simulink model "FS_AWD_Working"  (Simulink 10.0)
settings: Solver=ode45  StartTime=0.0  StopTime=inf  RelTol=1e-3  EnableMultiTasking=on
PreLoadFcn:
  | FSE_Parameters
undefined symbols (not defined in the file): i_Diff, TC_Decr_Gas, TC_Derivative, TC_Incr_Gas, TC_On, TC_Relay_Off, TC_Relay_On
libraries: CarMaker4SL x26, simulink x3, simulink_extras x2
(part 2 of 2)

== system FS_AWD_Working/CarMaker/IPG Vehicle/CarAndTrailer/Forces/Vehicle Forces ==
  Sync_In : Inport
  Bus Creator1 : BusCreator  Inputs=12
  Bus Creator8 : BusCreator  Inputs=16
  BusCreator1 : BusCreator  Inputs=4
  BusCreator2 : BusCreator  Inputs=9
  Demux : Demux  Outputs=16
  Demux1 : Demux  Outputs=12
  Demux2 : Demux  Outputs=13
  Forces : S-Function  FunctionName=CM_Sfun  Parameters='Forces'  SFunctionDeploymentMode=off  EnableBusSupport=off
  Terminator : Terminator
  Sync_Out : Outport  VectorParamsAs1DForOutWhenUnconnected=off
  Car.Virtual : Outport  Port=2  VectorParamsAs1DForOutWhenUnconnected=off
  Car.Aero : Outport  Port=3  VectorParamsAs1DForOutWhenUnconnected=off
  Car.Load : Outport  Port=4  VectorParamsAs1DForOutWhenUnconnected=off
  wires:
  BusCreator1/1 -> Terminator/1  "Aero IF (in)"
  Demux2/13 -> BusCreator2/9  "car Aero Trq_1 z"
  Demux2/12 -> BusCreator2/8  "car Aero Trq_1 y"
  Demux2/11 -> BusCreator2/7  "car Aero Trq_1 x"
  Demux2/10 -> BusCreator2/6  "car Aero Frc_1 z"
  Demux2/9 -> BusCreator2/5  "car Aero Frc_1 y"
  Demux2/8 -> BusCreator2/4  "car Aero Frc_1 x"
  Demux2/7 -> BusCreator2/3  "car Aero PoA_1 z"
  Demux2/6 -> BusCreator2/2  "car Aero PoA_1 y"
  Demux2/5 -> BusCreator2/1  "car Aero PoA_1 x"
  Demux2/4 -> BusCreator1/4  "car Aero tau_1"
  Demux2/3 -> BusCreator1/3  "car Aero ApproachVel_1 z"
  Demux2/2 -> BusCreator1/2  "car Aero ApproachVel_1 y"
  Demux2/1 -> BusCreator1/1  "car Aero ApproachVel_1 x"
  Demux/16 -> Bus Creator8/16  "Car Load_3 tz"
  Demux/15 -> Bus Creator8/15  "Car Load_3 ty"
  Demux/14 -> Bus Creator8/14  "Car Load_3 tx"
  Demux/13 -> Bus Creator8/13  "Car Load_3 mass"
  Demux1/12 -> Bus Creator1/12  "Car Virtual Trq_0 z"
  Demux1/11 -> Bus Creator1/11  "Car Virtual Trq_0 y"
  Demux1/10 -> Bus Creator1/10  "Car Virtual Trq_0 x"
  Demux1/9 -> Bus Creator1/9  "Car Virtual Trq_1 z"
  Demux1/8 -> Bus Creator1/8  "Car Virtual Trq_1 y"
  Demux1/7 -> Bus Creator1/7  "Car Virtual Trq_1 x"
  Demux1/6 -> Bus Creator1/6  "Car Virtual Frc_0 z"
  Demux1/5 -> Bus Creator1/5  "Car Virtual Frc_0 y"
  Demux1/4 -> Bus Creator1/4  "Car Virtual Frc_0 x"
  Sync_In/1 -> Forces/1
  Forces/1 -> Sync_Out/1
  BusCreator2/1 -> Car.Aero/1
  Demux1/1 -> Bus Creator1/1  "Car Virtual Frc_1 x"
  Demux1/2 -> Bus Creator1/2  "Car Virtual Frc_1 y"
  Demux1/3 -> Bus Creator1/3  "Car Virtual Frc_1 z"
  Forces/3 -> Demux2/1
  Forces/2 -> Demux1/1
  Bus Creator1/1 -> Car.Virtual/1
  Bus Creator8/1 -> Car.Load/1
  Demux/1 -> Bus Creator8/1  "Car Load_0 mass"
  Demux/2 -> Bus Creator8/2  "Car Load_0 tx"
  Demux/3 -> Bus Creator8/3  "Car Load_0 ty"
  Demux/4 -> Bus Creator8/4  "Car Load_0 tz"
  Demux/5 -> Bus Creator8/5  "Car Load_1 mass"
  Demux/6 -> Bus Creator8/6  "Car Load_1 tx"
  Demux/7 -> Bus Creator8/7  "Car Load_1 ty"
  Demux/8 -> Bus Creator8/8  "Car Load_1 tz"
  Demux/9 -> Bus Creator8/9  "Car Load_2 mass"
  Demux/10 -> Bus Creator8/10  "Car Load_2 tx"
  Demux/11 -> Bus Creator8/11  "Car Load_2 ty"
  Demux/12 -> Bus Creator8/12  "Car Load_2 tz"
  Forces/4 -> Demux/1

== system FS_AWD_Working/CarMaker/IPG Vehicle/CarAndTrailer/Trailer/CreateBus Car.Hitch.FrcTrq ==
  In1 : Inport
  Bus Creator7 : BusCreator  Inputs=6
  Demux7 : Demux  Outputs=6
  Out1 : Outport  VectorParamsAs1DForOutWhenUnconnected=off
  wires:
  In1/1 -> Demux7/1
  Bus Creator7/1 -> Out1/1
  Demux7/6 -> Bus Creator7/6  "Car Hitch Trq2Car z"
  Demux7/5 -> Bus Creator7/5  "Car Hitch Trq2Car y"
  Demux7/4 -> Bus Creator7/4  "Car Hitch Trq2Car x"
  Demux7/3 -> Bus Creator7/3  "Car Hitch Frc2Car z"
  Demux7/2 -> Bus Creator7/2  "Car Hitch Frc2Car y"
  Demux7/1 -> Bus Creator7/1  "Car Hitch Frc2Car x"

== system FS_AWD_Working/CarMaker/IPG Vehicle/CarAndTrailer/Trailer/CreateBus Vhcl.Motion ==
  In1 : Inport
  BusCreator : BusCreator  Inputs=15
  Demux : Demux  Outputs=15
  Out1 : Outport  VectorParamsAs1DForOutWhenUnconnected=off
  wires:
  Demux/15 -> BusCreator/15  "Vhcl YawAcc"
  Demux/14 -> BusCreator/14  "Vhcl YawVel"
  Demux/13 -> BusCreator/13  "Vhcl Yaw"
  Demux/12 -> BusCreator/12  "Vhcl PitchAcc"
  Demux/11 -> BusCreator/11  "Vhcl PitchVel"
  Demux/10 -> BusCreator/10  "Vhcl Pitch"
  Demux/9 -> BusCreator/9  "Vhcl RollAcc"
  Demux/8 -> BusCreator/8  "Vhcl RollVel"
  Demux/7 -> BusCreator/7  "Vhcl Roll"
  Demux/6 -> BusCreator/6  "Vhcl Hitch_Pos z"
  Demux/5 -> BusCreator/5  "Vhcl Hitch_Pos y"
  Demux/4 -> BusCreator/4  "Vhcl Hitch_Pos x"
  Demux/3 -> BusCreator/3  "Vhcl sRoad"
  Demux/2 -> BusCreator/2  "Vhcl Distance"
  Demux/1 -> BusCreator/1  "Vhcl v"
  In1/1 -> Demux/1
  BusCreator/1 -> Out1/1

== system FS_AWD_Working/CarMaker/IPG Vehicle/CarAndTrailer/Trailer/CreateBus Vhcl.PoI ==
  In1 : Inport
  Bus Creator3 : BusCreator  Inputs=18
  Demux3 : Demux  Outputs=18
  Out1 : Outport  VectorParamsAs1DForOutWhenUnconnected=off
  wires:
  Demux3/18 -> Bus Creator3/18  "Vhcl PoI_GCS Elev"
  Demux3/17 -> Bus Creator3/17  "Vhcl PoI_GCS Lat"
  Demux3/16 -> Bus Creator3/16  "Vhcl PoI_GCS Long"
  Demux3/15 -> Bus Creator3/15  "Vhcl PoI_Acc_1 z"
  Demux3/14 -> Bus Creator3/14  "Vhcl PoI_Acc_1 y"
  Demux3/13 -> Bus Creator3/13  "Vhcl PoI_Acc_1 x"
  Demux3/12 -> Bus Creator3/12  "Vhcl PoI_Vel_1 z"
  Demux3/11 -> Bus Creator3/11  "Vhcl PoI_Vel_1 y"
  Demux3/10 -> Bus Creator3/10  "Vhcl PoI_Vel_1 x"
  Demux3/9 -> Bus Creator3/9  "Vhcl PoI_Acc z"
  Demux3/8 -> Bus Creator3/8  "Vhcl PoI_Acc y"
  Demux3/7 -> Bus Creator3/7  "Vhcl PoI_Acc x"
  Demux3/6 -> Bus Creator3/6  "Vhcl PoI_Vel z"
  Demux3/5 -> Bus Creator3/5  "Vhcl PoI_Vel y"
  Demux3/4 -> Bus Creator3/4  "Vhcl PoI_Vel x"
  Demux3/3 -> Bus Creator3/3  "Vhcl PoI_Pos z"
  Demux3/2 -> Bus Creator3/2  "Vhcl PoI_Pos y"
  In1/1 -> Demux3/1
  Bus Creator3/1 -> Out1/1
  Demux3/1 -> Bus Creator3/1  "Vhcl PoI_Pos x"

== system FS_AWD_Working/CarMaker/IPG Vehicle/CarAndTrailer/Trailer/CreateBus Vhcl.Steering ==
  In1 : Inport
  Bus Creator3 : BusCreator  Inputs=4
  Demux : Demux
  Out1 : Outport  VectorParamsAs1DForOutWhenUnconnected=off
  wires:
  Bus Creator3/1 -> Out1/1
  Demux/1 -> Bus Creator3/1  "Vhcl Steering Ang"
  Demux/3 -> Bus Creator3/3  "Vhcl Steering AngAcc"
  Demux/2 -> Bus Creator3/2  "Vhcl Steering AngVel"
  Demux/4 -> Bus Creator3/4  "Vhcl Steering Trq"
  In1/1 -> Demux/1

== system FS_AWD_Working/CarMaker/IPG Vehicle/CarAndTrailer/Trailer/CreateBus Vhcl.Wheel.FL ==
  In1 : Inport
  Bus Creator3 : BusCreator  Inputs=14
  Demux3 : Demux  Outputs=14
  Out1 : Outport  VectorParamsAs1DForOutWhenUnconnected=off
  wires:
  Demux3/14 -> Bus Creator3/14  "Vhcl Wheel FL Trq_WhlBearing"
  Demux3/13 -> Bus Creator3/13  "Vhcl Wheel FL Trq_T2W"
  Demux3/12 -> Bus Creator3/12  "Vhcl Wheel FL SideSlip"
  Demux3/11 -> Bus Creator3/11  "Vhcl Wheel FL LongSlip"
  Demux3/10 -> Bus Creator3/10  "Vhcl Wheel FL vBelt"
  Demux3/9 -> Bus Creator3/9  "Vhcl Wheel FL Fz"
  Demux3/8 -> Bus Creator3/8  "Vhcl Wheel FL Fy"
  Demux3/7 -> Bus Creator3/7  "Vhcl Wheel FL Fx"
  Demux3/6 -> Bus Creator3/6  "Vhcl Wheel FL r_zxy z"
  Demux3/5 -> Bus Creator3/5  "Vhcl Wheel FL r_zxy y"
  Demux3/4 -> Bus Creator3/4  "Vhcl Wheel FL r_zxy x"
  Demux3/3 -> Bus Creator3/3  "Vhcl Wheel FL t z"
  Demux3/2 -> Bus Creator3/2  "Vhcl Wheel FL t y"
  In1/1 -> Demux3/1
  Bus Creator3/1 -> Out1/1
  Demux3/1 -> Bus Creator3/1  "Vhcl Wheel FL t x"

== system FS_AWD_Working/CarMaker/IPG Vehicle/CarAndTrailer/Trailer/CreateBus Vhcl.Wheel.FR ==
  In1 : Inport
  Bus Creator3 : BusCreator  Inputs=14
  Demux3 : Demux  Outputs=14
  Out1 : Outport  VectorParamsAs1DForOutWhenUnconnected=off
  wires:
  Demux3/14 -> Bus Creator3/14  "Vhcl Wheel FR Trq_WhlBearing"
  Demux3/13 -> Bus Creator3/13  "Vhcl Wheel FR Trq_T2W"
  Demux3/12 -> Bus Creator3/12  "Vhcl Wheel FR SideSlip"
  Demux3/11 -> Bus Creator3/11  "Vhcl Wheel FR LongSlip"
  Demux3/10 -> Bus Creator3/10  "Vhcl Wheel FR vBelt"
  Demux3/9 -> Bus Creator3/9  "Vhcl Wheel FR Fz"
  Demux3/8 -> Bus Creator3/8  "Vhcl Wheel FR Fy"
  Demux3/7 -> Bus Creator3/7  "Vhcl Wheel FR Fx"
  Demux3/6 -> Bus Creator3/6  "Vhcl Wheel FR r_zxy z"
  Demux3/5 -> Bus Creator3/5  "Vhcl Wheel FR r_zxy y"
  Demux3/4 -> Bus Creator3/4  "Vhcl Wheel FR r_zxy x"
  Demux3/3 -> Bus Creator3/3  "Vhcl Wheel FR t z"
  Demux3/2 -> Bus Creator3/2  "Vhcl Wheel FR t y"
  In1/1 -> Demux3/1
  Bus Creator3/1 -> Out1/1
  Demux3/1 -> Bus Creator3/1  "Vhcl Wheel FR t x"

== system FS_AWD_Working/CarMaker/IPG Vehicle/CarAndTrailer/Trailer/CreateBus Vhcl.Wheel.RL ==
  In1 : Inport
  Bus Creator3 : BusCreator  Inputs=14
  Demux3 : Demux  Outputs=14
  Out1 : Outport  VectorParamsAs1DForOutWhenUnconnected=off
  wires:
  Demux3/14 -> Bus Creator3/14  "Vhcl Wheel RL Trq_WhlBearing"
  Demux3/13 -> Bus Creator3/13  "Vhcl Wheel RL Trq_T2W"
  Demux3/12 -> Bus Creator3/12  "Vhcl Wheel RL SideSlip"
  Demux3/11 -> Bus Creator3/11  "Vhcl Wheel RL LongSlip"
  Demux3/10 -> Bus Creator3/10  "Vhcl Wheel RL vBelt"
  Demux3/9 -> Bus Creator3/9  "Vhcl Wheel RL Fz"
  Demux3/8 -> Bus Creator3/8  "Vhcl Wheel RL Fy"
  Demux3/7 -> Bus Creator3/7  "Vhcl Wheel RL Fx"
  Demux3/6 -> Bus Creator3/6  "Vhcl Wheel RL r_zxy z"
  Demux3/5 -> Bus Creator3/5  "Vhcl Wheel RL r_zxy y"
  Demux3/4 -> Bus Creator3/4  "Vhcl Wheel RL r_zxy x"
  Demux3/3 -> Bus Creator3/3  "Vhcl Wheel RL t z"
  Demux3/2 -> Bus Creator3/2  "Vhcl Wheel RL t y"
  In1/1 -> Demux3/1
  Bus Creator3/1 -> Out1/1
  Demux3/1 -> Bus Creator3/1  "Vhcl Wheel RL t x"

== system FS_AWD_Working/CarMaker/IPG Vehicle/CarAndTrailer/Trailer/CreateBus Vhcl.Wheel.RR ==
  In1 : Inport
  Bus Creator3 : BusCreator  Inputs=14
  Demux3 : Demux  Outputs=14
  Out1 : Outport  VectorParamsAs1DForOutWhenUnconnected=off
  wires:
  Demux3/14 -> Bus Creator3/14  "Vhcl Wheel RR Trq_WhlBearing"
  Demux3/13 -> Bus Creator3/13  "Vhcl Wheel RR Trq_T2W"
  Demux3/12 -> Bus Creator3/12  "Vhcl Wheel RR SideSlip"
  Demux3/11 -> Bus Creator3/11  "Vhcl Wheel RR LongSlip"
  Demux3/10 -> Bus Creator3/10  "Vhcl Wheel RR vBelt"
  Demux3/9 -> Bus Creator3/9  "Vhcl Wheel RR Fz"
  Demux3/8 -> Bus Creator3/8  "Vhcl Wheel RR Fy"
  Demux3/7 -> Bus Creator3/7  "Vhcl Wheel RR Fx"
  Demux3/6 -> Bus Creator3/6  "Vhcl Wheel RR r_zxy z"
  Demux3/5 -> Bus Creator3/5  "Vhcl Wheel RR r_zxy y"
  Demux3/4 -> Bus Creator3/4  "Vhcl Wheel RR r_zxy x"
  Demux3/3 -> Bus Creator3/3  "Vhcl Wheel RR t z"
  Demux3/2 -> Bus Creator3/2  "Vhcl Wheel RR t y"
  In1/1 -> Demux3/1
  Bus Creator3/1 -> Out1/1
  Demux3/1 -> Bus Creator3/1  "Vhcl Wheel RR t x"

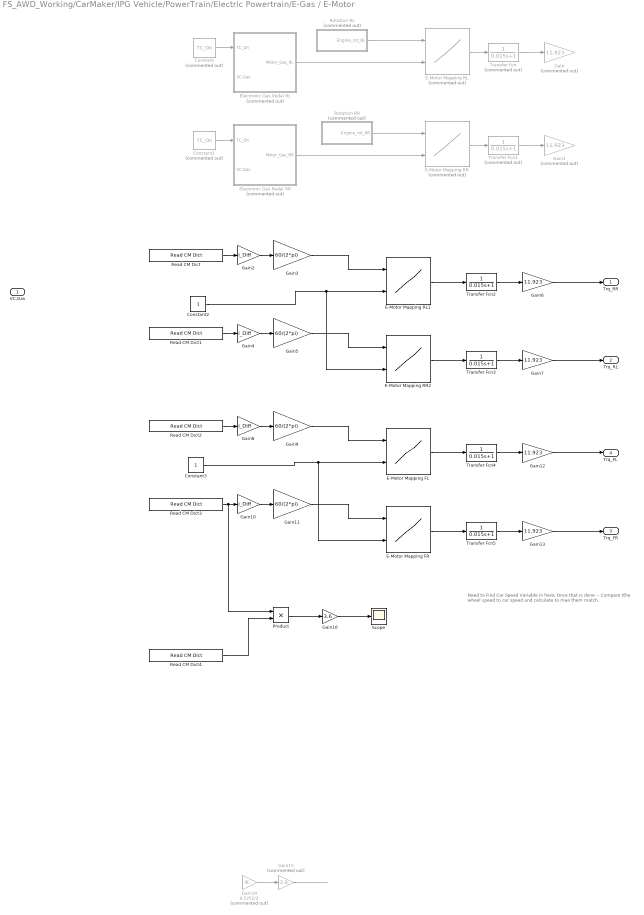
== system FS_AWD_Working/CarMaker/IPG Vehicle/PowerTrain/Electric Powertrain/E-Gas / E-Motor ==
  note: Need to Find Car Speed Variable in here;
      | Once that is done --
      | Compare tthe wheel speed to car speed and calculate to mae them match.
  VC.Gas : Inport
  Constant : Constant  Commented=on  Value=TC_On
  Constant1 : Constant  Commented=on  Value=TC_On
  Constant2 : Constant
  Constant3 : Constant
  E-Motor Mapping FL : Lookup2D  RowIndex=AMKData_GC(1,2:end)  ColumnIndex=AMKData_GC(2:end,1)  Table=AMKData_GC(2:end,2:end)'  LookUpMeth=Interpolation-Use End Values
  E-Motor Mapping FR : Lookup2D  RowIndex=AMKData_GC(1,2:end)  ColumnIndex=AMKData_GC(2:end,1)  Table=AMKData_GC(2:end,2:end)'  LookUpMeth=Interpolation-Use End Values
  E-Motor Mapping RL : Lookup2D  Commented=on  RowIndex=FSE_M120(1,2:end)  ColumnIndex=FSE_M120(2:end,1)  Table=FSE_M120(2:end,2:end)'  LookUpMeth=Interpolation-Use End Values
  E-Motor Mapping RL1 : Lookup2D  RowIndex=AMKData_GC(1,2:end)  ColumnIndex=AMKData_GC(2:end,1)  Table=AMKData_GC(2:end,2:end)'  LookUpMeth=Interpolation-Use End Values
  E-Motor Mapping RR : Lookup2D  Commented=on  RowIndex=FSE_M120(1,2:end)  ColumnIndex=FSE_M120(2:end,1)  Table=FSE_M120(2:end,2:end)'  LookUpMeth=Interpolation-Use End Values
  E-Motor Mapping RR2 : Lookup2D  RowIndex=AMKData_GC(1,2:end)  ColumnIndex=AMKData_GC(2:end,1)  Table=AMKData_GC(2:end,2:end)'  LookUpMeth=Interpolation-Use End Values
  Electronic Gas Pedal RL : Subsystem  Commented=on
  Electronic Gas Pedal RR : Subsystem  Commented=on
  Gain : Gain  Commented=on  Gain=11.923
  Gain1 : Gain  Commented=on  Gain=11.923
  Gain{2,4,8,10} (4 alike) : Gain  Gain=i_Diff
  Gain{3,5,9,11} (4 alike) : Gain  Gain=60/(2*pi)
  Gain{6..7,12..13} (4 alike) : Gain  Gain=11.923
  Gain14 : Gain  Commented=on  Gain=0.5252/2
  Gain15 : Gain  Commented=on  Gain=3.6
  Gain16 : Gain  Gain=3.6
  Product : Product
  Read CM Dict : CarMaker4SL/Read CM Dict  xname=Car.WheelSpd_RR  xsync=off
  Read CM Dict1 : CarMaker4SL/Read CM Dict  xname=Car.WheelSpd_RL  xsync=off
  Read CM Dict2 : CarMaker4SL/Read CM Dict  xname=Car.WheelSpd_FL  xsync=off
  Read CM Dict3 : CarMaker4SL/Read CM Dict  xname=Car.WheelSpd_FR  xsync=off
  Read CM Dict4 : CarMaker4SL/Read CM Dict  xname=Car.WFL.Radius  xsync=off
  Rotation RL : Subsystem  Commented=on
  Rotation RR : Subsystem  Commented=on
  Scope : Scope
  Transfer Fcn : TransferFcn  Commented=on  Denominator=[0.015 1]
  Transfer Fcn1 : TransferFcn  Commented=on  Denominator=[0.015 1]
  Transfer Fcn{2..5} (4 alike) : TransferFcn  Denominator=[0.015 1]
  Trq_RR : Outport  VectorParamsAs1DForOutWhenUnconnected=off
  Trq_RL : Outport  Port=2  VectorParamsAs1DForOutWhenUnconnected=off
  Trq_FR : Outport  Port=3  VectorParamsAs1DForOutWhenUnconnected=off
  Trq_FL : Outport  Port=4  VectorParamsAs1DForOutWhenUnconnected=off
  wires:
  Rotation RL/1(Engine_rot_RL) -> E-Motor Mapping RL/1
  Constant/1 -> Electronic Gas Pedal RL/1(TC_On)
  Electronic Gas Pedal RL/1(Motor_Gas_RL) -> E-Motor Mapping RL/2
  Constant1/1 -> Electronic Gas Pedal RR/1(TC_On)
  E-Motor Mapping RL/1 -> Transfer Fcn/1
  Transfer Fcn/1 -> Gain/1
  Rotation RR/1(Engine_rot_RR) -> E-Motor Mapping RR/1
  Electronic Gas Pedal RR/1(Motor_Gas_RR) -> E-Motor Mapping RR/2
  Transfer Fcn1/1 -> Gain1/1
  E-Motor Mapping RR/1 -> Transfer Fcn1/1
  Read CM Dict/1 -> Gain2/1
  Gain2/1 -> Gain3/1
  Gain3/1 -> E-Motor Mapping RL1/1
  Read CM Dict1/1 -> Gain4/1
  Gain4/1 -> Gain5/1
  Gain5/1 -> E-Motor Mapping RR2/1
  Transfer Fcn3/1 -> Gain7/1
  Transfer Fcn2/1 -> Gain6/1
  E-Motor Mapping RL1/1 -> Transfer Fcn2/1
  Gain6/1 -> Trq_RR/1
  Gain7/1 -> Trq_RL/1
  E-Motor Mapping RR2/1 -> Transfer Fcn3/1
  Gain9/1 -> E-Motor Mapping FL/1
  Transfer Fcn5/1 -> Gain13/1
  Transfer Fcn4/1 -> Gain12/1
  Gain12/1 -> Trq_FL/1
  Gain13/1 -> Trq_FR/1
  E-Motor Mapping FL/1 -> Transfer Fcn4/1
  Read CM Dict3/1 -> Product/1, Gain10/1
  Gain10/1 -> Gain11/1
  Gain8/1 -> Gain9/1
  E-Motor Mapping FR/1 -> Transfer Fcn5/1
  Read CM Dict2/1 -> Gain8/1
  Gain11/1 -> E-Motor Mapping FR/1
  Gain14/1 -> Gain15/1
  Gain15/1 -> ?
  Read CM Dict4/1 -> Product/2
  Product/1 -> Gain16/1
  Gain16/1 -> Scope/1
  Constant2/1 -> E-Motor Mapping RR2/2, E-Motor Mapping RL1/2
  Constant3/1 -> E-Motor Mapping FR/2, E-Motor Mapping FL/2

== system FS_AWD_Working/CarMaker/IPG Vehicle/PowerTrain/Electric Powertrain/Gas Pedal ==
  Clock : Clock
  Constant : Constant  Value=0
  Constant1 : Constant
  Fcn : Fcn  Commented=through  Expr=u==0
  Read CM Dict : CarMaker4SL/Read CM Dict  xname=Vhcl.Ignition  xsync=off
  Read CM Dict2 : CarMaker4SL/Read CM Dict  xname=VC.Gas  xsync=off
  Switch : Switch
  Switch1 : Switch
  Write CM Dict : CarMaker4SL/Write CM Dict  xname=Vhcl.Ignition  xsync=off
  VC.Gas : Outport  VectorParamsAs1DForOutWhenUnconnected=off
  wires:
  Read CM Dict2/1 -> Switch/1
  Switch/1 -> VC.Gas/1
  Constant/1 -> Switch/3
  Switch1/1 -> Switch/2, Write CM Dict/1
  Read CM Dict/1 -> Switch1/3
  Constant1/1 -> Switch1/1
  Fcn/1 -> Switch1/2
  Clock/1 -> Fcn/1

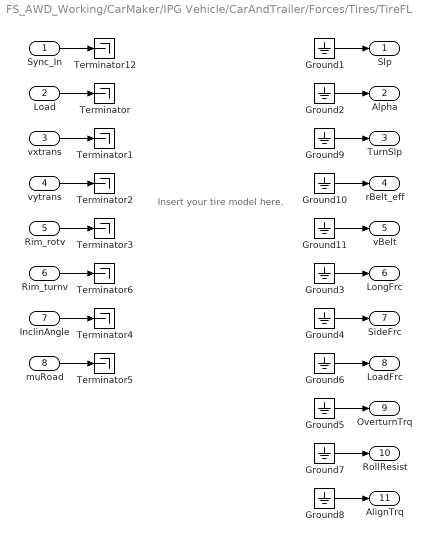
== system FS_AWD_Working/CarMaker/IPG Vehicle/CarAndTrailer/Forces/Tires/TireFL ==
  note: Insert your tire model here.
  Sync_In : Inport
  Load : Inport  Port=2
  vxtrans : Inport  Port=3
  vytrans : Inport  Port=4
  Rim_rotv : Inport  Port=5
  Rim_turnv : Inport  Port=6
  InclinAngle : Inport  Port=7
  muRoad : Inport  Port=8
  Ground{1..11} (11 alike) : Ground
  Terminator{,1..6,12} (8 alike) : Terminator
  Slp : Outport  VectorParamsAs1DForOutWhenUnconnected=off
  Alpha : Outport  Port=2  VectorParamsAs1DForOutWhenUnconnected=off
  TurnSlp : Outport  Port=3  VectorParamsAs1DForOutWhenUnconnected=off
  rBelt_eff : Outport  Port=4  VectorParamsAs1DForOutWhenUnconnected=off
  vBelt : Outport  Port=5  VectorParamsAs1DForOutWhenUnconnected=off
  LongFrc : Outport  Port=6  VectorParamsAs1DForOutWhenUnconnected=off
  SideFrc : Outport  Port=7  VectorParamsAs1DForOutWhenUnconnected=off
  LoadFrc : Outport  Port=8  VectorParamsAs1DForOutWhenUnconnected=off
  OverturnTrq : Outport  Port=9  VectorParamsAs1DForOutWhenUnconnected=off
  RollResist : Outport  Port=10  VectorParamsAs1DForOutWhenUnconnected=off
  AlignTrq : Outport  Port=11  VectorParamsAs1DForOutWhenUnconnected=off
  wires:
  Ground11/1 -> vBelt/1
  Ground10/1 -> rBelt_eff/1
  Ground9/1 -> TurnSlp/1
  Rim_turnv/1 -> Terminator6/1
  Sync_In/1 -> Terminator12/1
  Ground2/1 -> Alpha/1
  Ground3/1 -> LongFrc/1
  Ground4/1 -> SideFrc/1
  Ground5/1 -> OverturnTrq/1
  vxtrans/1 -> Terminator1/1
  vytrans/1 -> Terminator2/1
  Rim_rotv/1 -> Terminator3/1
  InclinAngle/1 -> Terminator4/1
  muRoad/1 -> Terminator5/1
  Load/1 -> Terminator/1
  Ground1/1 -> Slp/1
  Ground6/1 -> LoadFrc/1
  Ground7/1 -> RollResist/1
  Ground8/1 -> AlignTrq/1

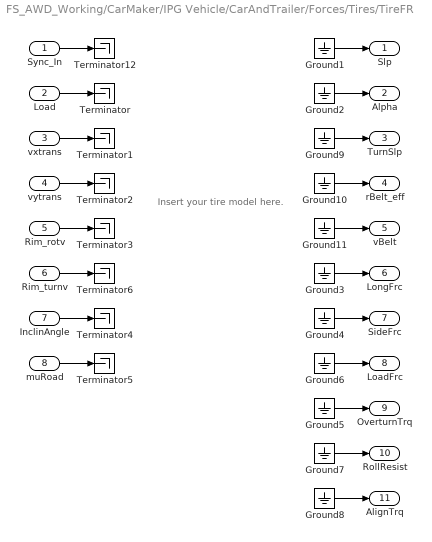
== system FS_AWD_Working/CarMaker/IPG Vehicle/CarAndTrailer/Forces/Tires/TireFR ==
  note: Insert your tire model here.
  Sync_In : Inport
  Load : Inport  Port=2
  vxtrans : Inport  Port=3
  vytrans : Inport  Port=4
  Rim_rotv : Inport  Port=5
  Rim_turnv : Inport  Port=6
  InclinAngle : Inport  Port=7
  muRoad : Inport  Port=8
  Ground{1..11} (11 alike) : Ground
  Terminator{,1..6,12} (8 alike) : Terminator
  Slp : Outport  VectorParamsAs1DForOutWhenUnconnected=off
  Alpha : Outport  Port=2  VectorParamsAs1DForOutWhenUnconnected=off
  TurnSlp : Outport  Port=3  VectorParamsAs1DForOutWhenUnconnected=off
  rBelt_eff : Outport  Port=4  VectorParamsAs1DForOutWhenUnconnected=off
  vBelt : Outport  Port=5  VectorParamsAs1DForOutWhenUnconnected=off
  LongFrc : Outport  Port=6  VectorParamsAs1DForOutWhenUnconnected=off
  SideFrc : Outport  Port=7  VectorParamsAs1DForOutWhenUnconnected=off
  LoadFrc : Outport  Port=8  VectorParamsAs1DForOutWhenUnconnected=off
  OverturnTrq : Outport  Port=9  VectorParamsAs1DForOutWhenUnconnected=off
  RollResist : Outport  Port=10  VectorParamsAs1DForOutWhenUnconnected=off
  AlignTrq : Outport  Port=11  VectorParamsAs1DForOutWhenUnconnected=off
  wires:
  Ground11/1 -> vBelt/1
  Ground10/1 -> rBelt_eff/1
  Ground9/1 -> TurnSlp/1
  Rim_turnv/1 -> Terminator6/1
  Sync_In/1 -> Terminator12/1
  Ground2/1 -> Alpha/1
  Ground3/1 -> LongFrc/1
  Ground4/1 -> SideFrc/1
  Ground5/1 -> OverturnTrq/1
  vxtrans/1 -> Terminator1/1
  vytrans/1 -> Terminator2/1
  Rim_rotv/1 -> Terminator3/1
  InclinAngle/1 -> Terminator4/1
  muRoad/1 -> Terminator5/1
  Load/1 -> Terminator/1
  Ground1/1 -> Slp/1
  Ground6/1 -> LoadFrc/1
  Ground7/1 -> RollResist/1
  Ground8/1 -> AlignTrq/1

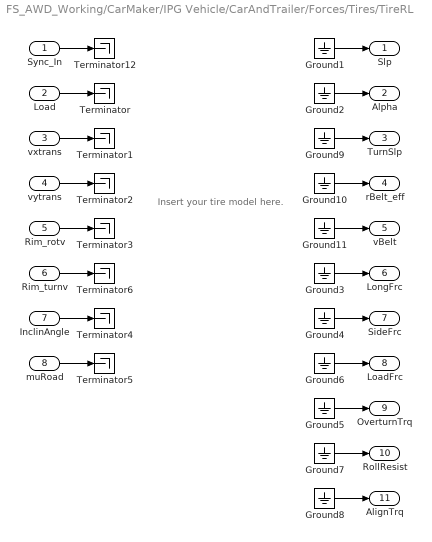
== system FS_AWD_Working/CarMaker/IPG Vehicle/CarAndTrailer/Forces/Tires/TireRL ==
  note: Insert your tire model here.
  Sync_In : Inport
  Load : Inport  Port=2
  vxtrans : Inport  Port=3
  vytrans : Inport  Port=4
  Rim_rotv : Inport  Port=5
  Rim_turnv : Inport  Port=6
  InclinAngle : Inport  Port=7
  muRoad : Inport  Port=8
  Ground{1..11} (11 alike) : Ground
  Terminator{,1..6,12} (8 alike) : Terminator
  Slp : Outport  VectorParamsAs1DForOutWhenUnconnected=off
  Alpha : Outport  Port=2  VectorParamsAs1DForOutWhenUnconnected=off
  TurnSlp : Outport  Port=3  VectorParamsAs1DForOutWhenUnconnected=off
  rBelt_eff : Outport  Port=4  VectorParamsAs1DForOutWhenUnconnected=off
  vBelt : Outport  Port=5  VectorParamsAs1DForOutWhenUnconnected=off
  LongFrc : Outport  Port=6  VectorParamsAs1DForOutWhenUnconnected=off
  SideFrc : Outport  Port=7  VectorParamsAs1DForOutWhenUnconnected=off
  LoadFrc : Outport  Port=8  VectorParamsAs1DForOutWhenUnconnected=off
  OverturnTrq : Outport  Port=9  VectorParamsAs1DForOutWhenUnconnected=off
  RollResist : Outport  Port=10  VectorParamsAs1DForOutWhenUnconnected=off
  AlignTrq : Outport  Port=11  VectorParamsAs1DForOutWhenUnconnected=off
  wires:
  Ground11/1 -> vBelt/1
  Ground10/1 -> rBelt_eff/1
  Ground9/1 -> TurnSlp/1
  Rim_turnv/1 -> Terminator6/1
  Sync_In/1 -> Terminator12/1
  Ground2/1 -> Alpha/1
  Ground3/1 -> LongFrc/1
  Ground4/1 -> SideFrc/1
  Ground5/1 -> OverturnTrq/1
  vxtrans/1 -> Terminator1/1
  vytrans/1 -> Terminator2/1
  Rim_rotv/1 -> Terminator3/1
  InclinAngle/1 -> Terminator4/1
  muRoad/1 -> Terminator5/1
  Load/1 -> Terminator/1
  Ground1/1 -> Slp/1
  Ground6/1 -> LoadFrc/1
  Ground7/1 -> RollResist/1
  Ground8/1 -> AlignTrq/1

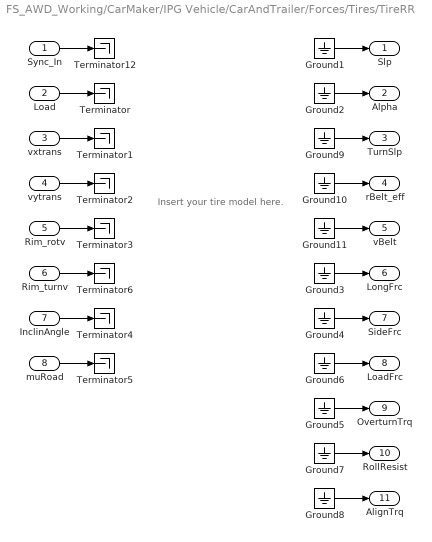
== system FS_AWD_Working/CarMaker/IPG Vehicle/CarAndTrailer/Forces/Tires/TireRR ==
  note: Insert your tire model here.
  Sync_In : Inport
  Load : Inport  Port=2
  vxtrans : Inport  Port=3
  vytrans : Inport  Port=4
  Rim_rotv : Inport  Port=5
  Rim_turnv : Inport  Port=6
  InclinAngle : Inport  Port=7
  muRoad : Inport  Port=8
  Ground{1..11} (11 alike) : Ground
  Terminator{,1..6,12} (8 alike) : Terminator
  Slp : Outport  VectorParamsAs1DForOutWhenUnconnected=off
  Alpha : Outport  Port=2  VectorParamsAs1DForOutWhenUnconnected=off
  TurnSlp : Outport  Port=3  VectorParamsAs1DForOutWhenUnconnected=off
  rBelt_eff : Outport  Port=4  VectorParamsAs1DForOutWhenUnconnected=off
  vBelt : Outport  Port=5  VectorParamsAs1DForOutWhenUnconnected=off
  LongFrc : Outport  Port=6  VectorParamsAs1DForOutWhenUnconnected=off
  SideFrc : Outport  Port=7  VectorParamsAs1DForOutWhenUnconnected=off
  LoadFrc : Outport  Port=8  VectorParamsAs1DForOutWhenUnconnected=off
  OverturnTrq : Outport  Port=9  VectorParamsAs1DForOutWhenUnconnected=off
  RollResist : Outport  Port=10  VectorParamsAs1DForOutWhenUnconnected=off
  AlignTrq : Outport  Port=11  VectorParamsAs1DForOutWhenUnconnected=off
  wires:
  Ground11/1 -> vBelt/1
  Ground10/1 -> rBelt_eff/1
  Ground9/1 -> TurnSlp/1
  Rim_turnv/1 -> Terminator6/1
  Sync_In/1 -> Terminator12/1
  Ground2/1 -> Alpha/1
  Ground3/1 -> LongFrc/1
  Ground4/1 -> SideFrc/1
  Ground5/1 -> OverturnTrq/1
  vxtrans/1 -> Terminator1/1
  vytrans/1 -> Terminator2/1
  Rim_rotv/1 -> Terminator3/1
  InclinAngle/1 -> Terminator4/1
  muRoad/1 -> Terminator5/1
  Load/1 -> Terminator/1
  Ground1/1 -> Slp/1
  Ground6/1 -> LoadFrc/1
  Ground7/1 -> RollResist/1
  Ground8/1 -> AlignTrq/1

== system FS_AWD_Working/CarMaker/IPG Vehicle/PowerTrain/Electric Powertrain/E-Gas / E-Motor/Electronic Gas Pedal RL ==
  TC_On : Inport
  VC.Gas : Inport  Port=2
  Define CM Dict : CarMaker4SL/Define CM Dict  xname=E_Gas_RL  xmono=off  xtype=Double4  xdvaplace=None  xnstates=0  xfirststate=0  xinitial=0
  Read CM Dict1 : CarMaker4SL/Read CM Dict  xname=E_Gas_RL  xsync=off
  Read CM Dict2 : CarMaker4SL/Read CM Dict  xname=Car.LongSlipRL  xsync=off
  Scope : Scope
  Subsystem1 : Subsystem
  Switch : Switch
  Write CM Dict : CarMaker4SL/Write CM Dict  xname=E_Gas_RL  xsync=off
  Motor_Gas_RL : Outport  VectorParamsAs1DForOutWhenUnconnected=off
  wires:
  VC.Gas/1 -> Switch/3, Subsystem1/1(VC.Gas)
  Switch/1 -> Motor_Gas_RL/1
  TC_On/1 -> Switch/2
  Subsystem1/1(E_Gas) -> Write CM Dict/1, Switch/1
  Read CM Dict1/1 -> Subsystem1/2(E_Gas.)
  Read CM Dict2/1 -> Scope/1, Subsystem1/3(Car.LongSlip)

== system FS_AWD_Working/CarMaker/IPG Vehicle/PowerTrain/Electric Powertrain/E-Gas / E-Motor/Electronic Gas Pedal RR ==
  TC_On : Inport
  VC.Gas : Inport  Port=2
  Define CM Dict : CarMaker4SL/Define CM Dict  xname=E_Gas_RR  xmono=off  xtype=Double4  xdvaplace=None  xnstates=0  xfirststate=0  xinitial=0
  Read CM Dict1 : CarMaker4SL/Read CM Dict  xname=E_Gas_RR  xsync=off
  Read CM Dict2 : CarMaker4SL/Read CM Dict  xname=Car.LongSlipRR  xsync=off
  Subsystem1 : Subsystem
  Switch : Switch
  Write CM Dict : CarMaker4SL/Write CM Dict  xname=E_Gas_RR  xsync=off
  Motor_Gas_RR : Outport  VectorParamsAs1DForOutWhenUnconnected=off
  wires:
  TC_On/1 -> Switch/2
  Switch/1 -> Motor_Gas_RR/1
  VC.Gas/1 -> Switch/3, Subsystem1/1(VC.Gas)
  Subsystem1/1(E_Gas) -> Write CM Dict/1, Switch/1
  Read CM Dict2/1 -> Subsystem1/3(Car.LongSlip)
  Read CM Dict1/1 -> Subsystem1/2(E_Gas.)

== system FS_AWD_Working/CarMaker/IPG Vehicle/PowerTrain/Electric Powertrain/E-Gas / E-Motor/Rotation RL ==
  Gain : Gain  Gain=i_Diff
  Gain1 : Gain  Gain=60/(2*pi)
  Read CM Dict : CarMaker4SL/Read CM Dict  xname=Car.WheelSpd_RL  xsync=off
  Engine_rot_RL : Outport  VectorParamsAs1DForOutWhenUnconnected=off
  wires:
  Read CM Dict/1 -> Gain/1
  Gain/1 -> Gain1/1
  Gain1/1 -> Engine_rot_RL/1

== system FS_AWD_Working/CarMaker/IPG Vehicle/PowerTrain/Electric Powertrain/E-Gas / E-Motor/Rotation RR ==
  Gain : Gain  Gain=i_Diff
  Gain1 : Gain  Gain=60/(2*pi)
  Read CM Dict : CarMaker4SL/Read CM Dict  xname=Car.WheelSpd_RR  xsync=off
  Engine_rot_RR : Outport  VectorParamsAs1DForOutWhenUnconnected=off
  wires:
  Gain1/1 -> Engine_rot_RR/1
  Gain/1 -> Gain1/1
  Read CM Dict/1 -> Gain/1

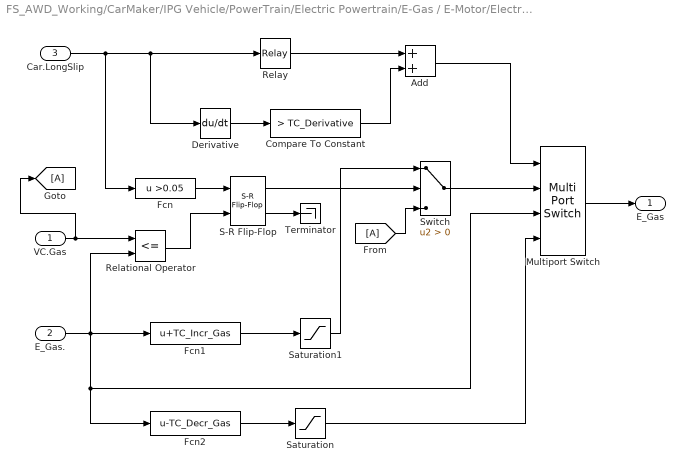
== system FS_AWD_Working/CarMaker/IPG Vehicle/PowerTrain/Electric Powertrain/E-Gas / E-Motor/Electronic Gas Pedal RL/Subsystem1 ==
  VC.Gas : Inport
  E_Gas. : Inport  Port=2
  Car.LongSlip : Inport  Port=3
  Add : Sum
  Compare To Constant : simulink/Logic and Bit Operations/Compare To Constant  relop=>  const=TC_Derivative  OutDataTypeStr=uint8  ZeroCross=off
  Derivative : Derivative
  Fcn : Fcn  Expr=u >0.05
  Fcn1 : Fcn  Expr=u+TC_Incr_Gas
  Fcn2 : Fcn  Expr=u-TC_Decr_Gas
  Multiport Switch : MultiPortSwitch  DataPortOrder=Zero-based contiguous  zeroidx=on
  Relational Operator : RelationalOperator  Operator=<=  RndMeth=Nearest
  Relay : Relay  OnSwitchValue=TC_Relay_On  OffSwitchValue=TC_Relay_Off
  S-R Flip-Flop : simulink_extras/Flip Flops/S-R Flip-Flop  initial_condition=0
  Saturation : Saturate  UpperLimit=1  LowerLimit=0
  Saturation1 : Saturate  UpperLimit=1  LowerLimit=0
  Switch : Switch  Criteria=u2 > Threshold
  Terminator : Terminator
  E_Gas : Outport  VectorParamsAs1DForOutWhenUnconnected=off
  wires:
  Car.LongSlip/1 -> Relay/1, Derivative/1, Fcn/1
  Relay/1 -> Add/1
  Derivative/1 -> Compare To Constant/1
  Compare To Constant/1 -> Add/2
  Add/1 -> Multiport Switch/1
  Multiport Switch/1 -> E_Gas/1
  VC.Gas/1 -> Relational Operator/1, [A]
  E_Gas./1 -> Relational Operator/2, Fcn1/1, Fcn2/1, Multiport Switch/3
  S-R Flip-Flop/2 -> Terminator/1
  S-R Flip-Flop/1 -> Switch/2
  Switch/1 -> Multiport Switch/2
  Fcn/1 -> S-R Flip-Flop/1
  Relational Operator/1 -> S-R Flip-Flop/2
  Fcn1/1 -> Saturation1/1
  Saturation1/1 -> Switch/1
  Fcn2/1 -> Saturation/1
  Saturation/1 -> Multiport Switch/4
  [A] -> Switch/3

== system FS_AWD_Working/CarMaker/IPG Vehicle/PowerTrain/Electric Powertrain/E-Gas / E-Motor/Electronic Gas Pedal RR/Subsystem1 ==
  VC.Gas : Inport
  E_Gas. : Inport  Port=2
  Car.LongSlip : Inport  Port=3
  Add : Sum
  Compare To Constant : simulink/Logic and Bit Operations/Compare To Constant  relop=>  const=TC_Derivative  OutDataTypeStr=uint8  ZeroCross=off
  Derivative : Derivative
  Fcn : Fcn  Expr=u >0.05
  Fcn1 : Fcn  Expr=u+TC_Incr_Gas
  Fcn2 : Fcn  Expr=u-TC_Decr_Gas
  Multiport Switch : MultiPortSwitch  DataPortOrder=Zero-based contiguous  zeroidx=on
  Relational Operator : RelationalOperator  Operator=<=  RndMeth=Nearest  InputSameDT=on
  Relay : Relay  OnSwitchValue=TC_Relay_On  OffSwitchValue=TC_Relay_Off
  S-R Flip-Flop : simulink_extras/Flip Flops/S-R Flip-Flop  initial_condition=0
  Saturation : Saturate  UpperLimit=1  LowerLimit=0
  Saturation1 : Saturate  UpperLimit=1  LowerLimit=0
  Switch : Switch  Criteria=u2 > Threshold
  Terminator : Terminator
  E_Gas : Outport  VectorParamsAs1DForOutWhenUnconnected=off
  wires:
  Car.LongSlip/1 -> Relay/1, Derivative/1, Fcn/1
  Relay/1 -> Add/1
  Derivative/1 -> Compare To Constant/1
  Compare To Constant/1 -> Add/2
  Add/1 -> Multiport Switch/1
  Multiport Switch/1 -> E_Gas/1
  VC.Gas/1 -> Relational Operator/1, [A]
  E_Gas./1 -> Relational Operator/2, Fcn1/1, Fcn2/1, Multiport Switch/3
  S-R Flip-Flop/2 -> Terminator/1
  S-R Flip-Flop/1 -> Switch/2
  Switch/1 -> Multiport Switch/2
  Fcn/1 -> S-R Flip-Flop/1
  Relational Operator/1 -> S-R Flip-Flop/2
  Fcn1/1 -> Saturation1/1
  Saturation1/1 -> Switch/1
  Fcn2/1 -> Saturation/1
  Saturation/1 -> Multiport Switch/4
  [A] -> Switch/3
